simulink model "WECSminiProject1"  (R2017b)
settings: Solver=ode45  StartTime=0.0  StopTime=1  MaxStep=1e-4  RelTol=1e-4  EnableMultiTasking=on
values from neighbouring files (symbols this model uses):
  Lm = 2.1346*10^(-3)    (= 0.0021346)    [WECSConstants.m]
  Lr = (0.06492*10^(-3)) + (2.1346*10^(-3))    (= 0.00219952)    [WECSConstants.m]
  Ls = (0.06492*10^(-3)) + (2.1346*10^(-3))    (= 0.00219952)    [WECSConstants.m]
libraries: powerlib x8
settings Model: Creator=Waseem  LastModifiedBy=zee_waqar
settings OptimizationCC: LifeSpan=inf
settings DebuggingCC: SFUnexpectedBacktrackingDiag=warning  SFNoUnconditionalDefaultTransitionDiag=warning  SFExecutionAtInitializationDiag=none
settings CodeAppCC: StateflowObjectComments=on
settings GRTTargetCC: TargetLangStandard=C89/C90 (ANSI)  GeneratePreprocessorConditionals=Disable all
settings ConfigComp: CovMetricSettings=dw  CovHtmlReporting=on  CovSaveCumulativeToWorkspaceVar=on  CovSaveSingleToWorkspaceVar=on  CovExternalEMLEnable=off
settings SimscapeCC: SimscapeNormalizeSystem=off

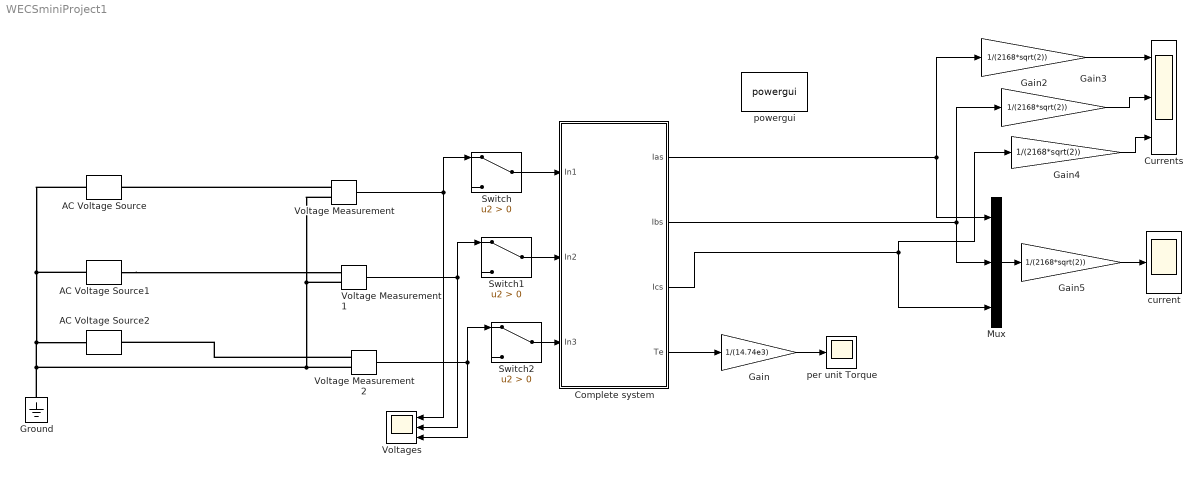
== system WECSminiProject1 ==
  AC Voltage Source : powerlib/Electrical Sources/AC Voltage Source  Amplitude=975.80  Phase=0  Frequency=50  SampleTime=1e-6  Measurements=Voltage  BusType=PV  Pref=2.30e6  Qref=0  Qmin=-inf  Qmax=+inf
  AC Voltage Source1 : powerlib/Electrical Sources/AC Voltage Source  Amplitude=975.80  Phase=120  Frequency=50  SampleTime=1e-6  Measurements=Voltage  BusType=PV  Pref=2.30e6  Qref=0  Qmin=-inf  Qmax=+inf
  AC Voltage Source2 : powerlib/Electrical Sources/AC Voltage Source  Amplitude=975.80  Phase=240  Frequency=50  SampleTime=1e-6  Measurements=Voltage  BusType=PV  Pref=2.30e6  Qref=0  Qmin=-inf  Qmax=+inf
  Complete system : Subsystem
  Currents : Scope  NumInputPorts=3
  Gain : Gain  Gain=1/(14.74e3)
  Gain{2..5} (4 alike) : Gain  Gain=1/(2168*sqrt(2))
  Ground : powerlib/Elements/Ground  LConnTagsString=a
  Mux : Mux  Inputs=3
  Switch : Switch  Criteria=u2 > Threshold
  Switch1 : Switch  Criteria=u2 > Threshold
  Switch2 : Switch  Criteria=u2 > Threshold
  Voltage Measurement : powerlib/Measurements/Voltage Measurement  PhasorSimulation=off  OutputType=Complex  PSBequivalent=0
  Voltage Measurement1 : powerlib/Measurements/Voltage Measurement  PhasorSimulation=off  OutputType=Complex  PSBequivalent=0
  Voltage Measurement2 : powerlib/Measurements/Voltage Measurement  PhasorSimulation=off  OutputType=Complex  PSBequivalent=0
  Voltages : Scope  NumInputPorts=3
  current : Scope
  per unit Torque : Scope
  powergui : powerlib/powergui  Priority=1  SimulationMode=Continuous  SampleTime=50e-6  frequency=60  Iterations=50  frequencyindice=50  Pbase=100e6  ErrMax=1e-4  UnitsV=kV  UnitsW=MW  buscounter=0  FunctionMessages=off  echomessages=off  EnableUseOfTLC=off  CurrentSourceSwitches=on  DisableSnubberDevices=off  DisableRonSwitches=off  DisableVfSwitches=off  DisplayEquations=off  SolverType=Tustin  Interpol=off  ExternalGateDelay=off  methode=off  Ts=10  x0status=blocks  SPID=off  SwTol=0  HookPort=off  RestoreLinks=warning  ResistiveCurrentMeasurement=off  Frange=[0:2:500]  Ylog=off  Xlog=on  ShowGrid=off  save=off  variable=ZData  structure=0  ZoomFFT=off  StartTime=0.0  cycles=1  DisplayStyle=1  fundamental=60  FreqAxis=off  MaxFrequency=1000  frequencyindicesteady=1  RmsSteady=1  display=off
  wires:
  Mux/1 -> Gain5/1
  Complete system/2(Ibs) -> Gain3/1, Mux/2
  Complete system/3(Ics) -> Mux/3, Gain4/1
  Complete system/1(Ias) -> Gain2/1, Mux/1
  Gain/1 -> per unit Torque/1
  Complete system/4(Te) -> Gain/1
  Gain2/1 -> Currents/1
  Gain3/1 -> Currents/2
  Gain4/1 -> Currents/3
  Gain5/1 -> current/1
  Voltage Measurement/1 -> Switch/1, Voltages/1
  Voltage Measurement1/1 -> Switch1/1, Voltages/2
  Voltage Measurement2/1 -> Switch2/1, Voltages/3
  Switch/1 -> Complete system/1(In1)
  Switch1/1 -> Complete system/2(In2)
  Switch2/1 -> Complete system/3(In3)
  connections:
  Ground/LConn1 -- Voltage Measurement/LConn2 -- Voltage Measurement1/LConn2 -- Voltage Measurement2/LConn2 -- AC Voltage Source/LConn1 -- AC Voltage Source1/LConn1 -- AC Voltage Source2/LConn1
  Voltage Measurement/LConn1 -- AC Voltage Source/RConn1
  AC Voltage Source1/RConn1 -- Voltage Measurement1/LConn1
  Voltage Measurement2/LConn1 -- AC Voltage Source2/RConn1

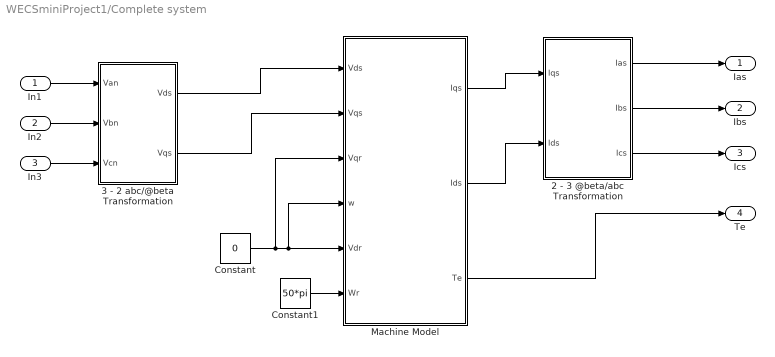
== system WECSminiProject1/Complete system ==
  In1 : Inport
  In2 : Inport  Port=2
  In3 : Inport  Port=3
  2 - 3 @beta/abc Transformation : Subsystem
  3 - 2 abc/@beta Transformation : Subsystem
  Constant : Constant  Value=0
  Constant1 : Constant  Value=50*pi
  Machine Model : Subsystem  mask{P=2, Rs=1.102e-3, Rr=1.497e-3, Ls=(0.06492e-3) + (2.1346e-3), Lr=(0.06492e-3) + (2.1346e-3), Lm=2.1346e-3, J=1200, D1=(Ls*Lr) - (Lm.^2), Tm=14.74* 10^3}
  Ias : Outport
  Ibs : Outport  Port=2
  Ics : Outport  Port=3
  Te : Outport  Port=4
  wires:
  2 - 3 @beta/abc Transformation/2(Ibs) -> Ibs/1
  2 - 3 @beta/abc Transformation/3(Ics) -> Ics/1
  2 - 3 @beta/abc Transformation/1(Ias) -> Ias/1
  Constant/1 -> Machine Model/3(Vqr), Machine Model/4(w), Machine Model/5(Vdr)
  Machine Model/1(Iqs) -> 2 - 3 @beta/abc Transformation/1(Iqs)
  3 - 2 abc/@beta Transformation/1(Vds) -> Machine Model/1(Vds)
  Machine Model/2(Ids) -> 2 - 3 @beta/abc Transformation/2(Ids)
  3 - 2 abc/@beta Transformation/2(Vqs) -> Machine Model/2("Vqs ")
  Machine Model/3(Te) -> Te/1
  In2/1 -> 3 - 2 abc/@beta Transformation/2(Vbn)
  In1/1 -> 3 - 2 abc/@beta Transformation/1(Van)
  In3/1 -> 3 - 2 abc/@beta Transformation/3(Vcn)
  Constant1/1 -> Machine Model/6(Wr)

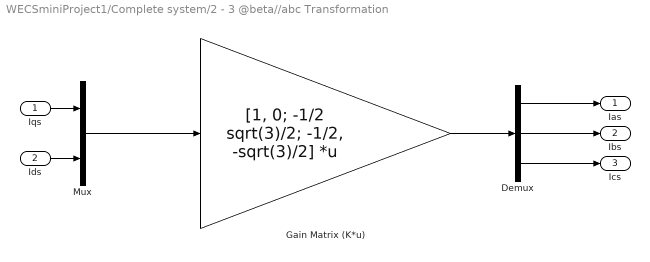
== system WECSminiProject1/Complete system/2 - 3 @beta//abc Transformation ==
  Iqs : Inport
  Ids : Inport  Port=2
  Demux : Demux  Outputs=3
  Gain Matrix (K*u) : Gain  Gain=[1, 0; -1/2 sqrt(3)/2; -1/2, -sqrt(3)/2]  Multiplication=Matrix(K*u)
  Mux : Mux  Inputs=2
  Ias : Outport
  Ibs : Outport  Port=2
  Ics : Outport  Port=3
  wires:
  Mux/1 -> Gain Matrix (K*u)/1
  Gain Matrix (K*u)/1 -> Demux/1
  Demux/2 -> Ibs/1
  Demux/1 -> Ias/1
  Demux/3 -> Ics/1
  Iqs/1 -> Mux/1
  Ids/1 -> Mux/2

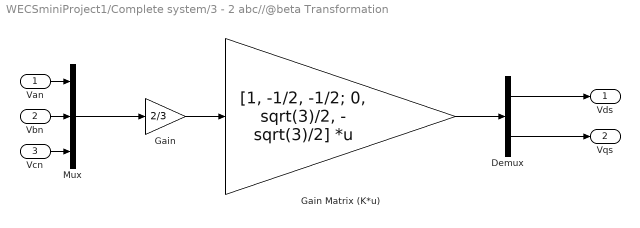
== system WECSminiProject1/Complete system/3 - 2 abc//@beta Transformation ==
  Van : Inport
  Vbn : Inport  Port=2
  Vcn : Inport  Port=3
  Demux : Demux  Outputs=2
  Gain : Gain  Gain=2/3
  Gain Matrix (K*u) : Gain  Gain=[1, -1/2, -1/2; 0, sqrt(3)/2, - sqrt(3)/2]  Multiplication=Matrix(K*u)
  Mux : Mux  Inputs=3
  Vds : Outport
  Vqs : Outport  Port=2
  wires:
  Vcn/1 -> Mux/3
  Vbn/1 -> Mux/2
  Van/1 -> Mux/1
  Gain/1 -> Gain Matrix (K*u)/1
  Gain Matrix (K*u)/1 -> Demux/1
  Mux/1 -> Gain/1
  Demux/1 -> Vds/1
  Demux/2 -> Vqs/1

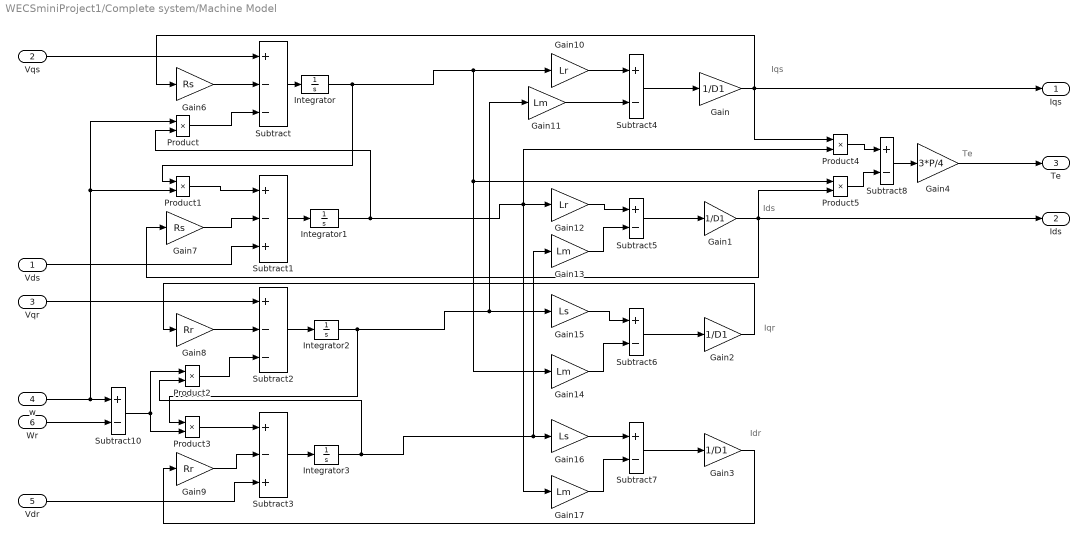
== system WECSminiProject1/Complete system/Machine Model ==
  note: Idr
  note: Iqr
  note: Te
  note: Ids
  note: Iqs
  Vds : Inport
  "Vqs " : Inport  Port=2
  Vqr : Inport  Port=3
  w : Inport  Port=4
  Vdr : Inport  Port=5
  Wr : Inport  Port=6
  Gain{,1..3} (4 alike) : Gain  Gain=1/D1
  Gain10 : Gain  Gain=Lr
  Gain{11,13..14,17} (4 alike) : Gain  Gain=Lm
  Gain12 : Gain  Gain=Lr
  Gain15 : Gain  Gain=Ls
  Gain16 : Gain  Gain=Ls
  Gain4 : Gain  Gain=3*P/4
  Gain6 : Gain  Gain=Rs
  Gain7 : Gain  Gain=Rs
  Gain8 : Gain  Gain=Rr
  Gain9 : Gain  Gain=Rr
  Integrator : Integrator  InitialCondition=1.79
  Integrator1 : Integrator  InitialCondition=1.79
  Integrator2 : Integrator  InitialCondition=1.70
  Integrator3 : Integrator  InitialCondition=1.70
  Product{,1..5} (6 alike) : Product
  Subtract : Sum  Inputs=+--
  Subtract1 : Sum  Inputs=+-+
  Subtract{4..8,10} (6 alike) : Sum  Inputs=+-
  Subtract2 : Sum  Inputs=+--
  Subtract3 : Sum  Inputs=+-+
  Iqs : Outport
  Ids : Outport  Port=2
  Te : Outport  Port=3
  wires:
  Subtract/1 -> Integrator/1
  Integrator/1 -> Gain10/1, Product5/1, Gain14/1, Product1/1
  Subtract1/1 -> Integrator1/1
  Subtract2/1 -> Integrator2/1
  Subtract3/1 -> Integrator3/1
  Subtract4/1 -> Gain/1
  Subtract5/1 -> Gain1/1
  Subtract6/1 -> Gain2/1
  Subtract7/1 -> Gain3/1
  Subtract8/1 -> Gain4/1
  Product4/1 -> Subtract8/1
  Gain/1 -> Product4/1, Iqs/1, Gain6/1
  Gain10/1 -> Subtract4/1
  Gain11/1 -> Subtract4/2
  Gain6/1 -> Subtract/2
  Product/1 -> Subtract/3
  Product1/1 -> Subtract1/1
  Gain7/1 -> Subtract1/2
  w/1 -> Subtract10/1, Product1/2, Product/1
  Gain12/1 -> Subtract5/1
  Gain13/1 -> Subtract5/2
  Integrator1/1 -> Product/2, Product4/2, Gain17/1, Gain12/1
  Gain1/1 -> Gain7/1, Ids/1, Product5/2
  Product5/1 -> Subtract8/2
  Gain4/1 -> Te/1
  Gain8/1 -> Subtract2/2
  Product2/1 -> Subtract2/3
  Vqr/1 -> Subtract2/1
  Gain14/1 -> Subtract6/2
  Gain15/1 -> Subtract6/1
  Integrator2/1 -> Gain11/1, Gain15/1, Product3/1
  Gain2/1 -> Gain8/1
  Subtract10/1 -> Product3/2, Product2/1
  Product3/1 -> Subtract3/1
  Gain9/1 -> Subtract3/2
  Integrator3/1 -> Product2/2, Gain13/1, Gain16/1
  Gain16/1 -> Subtract7/1
  Gain17/1 -> Subtract7/2
  Gain3/1 -> Gain9/1
  Vdr/1 -> Subtract3/3
  Vds/1 -> Subtract1/3
  "Vqs "/1 -> Subtract/1
  Wr/1 -> Subtract10/2
